simulink model "problem__8"  (R2020b)
settings: Solver=VariableStepAuto  StartTime=0.0  StopTime=10.0  RelTol=1e-3
settings Model: Creator=hp  LastModifiedBy=hp

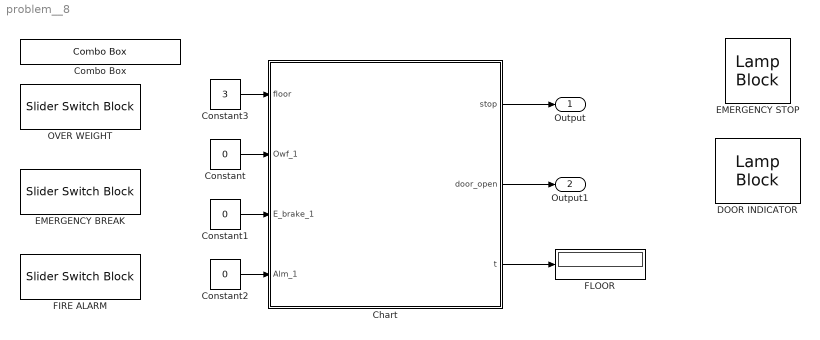
== system problem__8 ==
  Chart : Stateflow chart  TreatAsAtomicUnit=on
  Combo Box : ComboBox  LabelPosition=Hide  SelectedLabel=3rd FLOOR
      settings: Values={{'GROUND FLOOR', '1st FLOOR', '2nd FLOOR', '3rd FLOOR', '4thFLOOR'}, [0 1 2 3 4]}
  Constant : Constant  Value=0
  Constant1 : Constant  Value=0
  Constant2 : Constant  Value=0
  Constant3 : Constant  Value=3
  DOOR INDICATOR : LampBlock
  EMERGENCY BREAK : SliderSwitchBlock
      settings: Values={{'Off', 'On'}, [0 1]}
  EMERGENCY STOP : LampBlock
  FIRE ALARM : SliderSwitchBlock
      settings: Values={{'Off', 'On'}, [0 1]}
  "FLOOR " : Display
  OVER WEIGHT : SliderSwitchBlock
      settings: Values={{'Off', 'On'}, [0 1]}
  Output : Outport
  Output1 : Outport  Port=2
  wires:
  Chart/1(stop) -> Output/1
  Chart/2(door_open) -> Output1/1
  Chart/3(t) -> "FLOOR "/1
  Constant2/1 -> Chart/4(Alm_1)
  Constant/1 -> Chart/2(Owf_1)
  Constant1/1 -> Chart/3(E_brake_1)
  Constant3/1 -> Chart/1(floor)

== stateflow chart problem__8/Chart ==
  state overweight_flag(owf_1) [function]
    (default) -> (junction 160)
    (junction 160) -> (junction 162) [order 1] : [owf_1 ==1]
    (junction 160) -> (junction 167) [order 2]
    (junction 162) -> (junction 165) : {stop=1;}
    (junction 165) -> (junction 167)
    (junction 167) -> (junction 170)
  state LIFT_CONTROL
    state CONTROL
      en:
      i=0;
      i=floor;
      door_open=0;
      overweight_flag(Owf_1);
      fire_alarm(Alm_1);
      emergency_brake(E_brake_1);
      door_open=0;
    state FIRST
      en:
      i=1;
      door_open=1;
      t=1;
      ex:
      door_open=0;
    state SECOND
      en:
      i=2;
      door_open=1;
      t=2;
      ex:
      door_open=0;
    state THIRD
      en:
      i=3;
      door_open=1;
      t=3
      ex:
      door_open=0;
    state FOURTH
      en:
      i=4;
      door_open=1;
      t=4;
      ex:
      door_open=0;
    state GROUND
      en:
      i=0;
      door_open=1;
      t=0;
      ex:
      door_open=0;
    CONTROL -> FOURTH [order 5] : [i==4]
    CONTROL -> THIRD [order 4] : [i==3]
    CONTROL -> SECOND [order 3] : [i==2]
    CONTROL -> FIRST [order 2] : [i==1]
    (default) -> CONTROL
    CONTROL -> GROUND [order 1] : [i==0]
    SECOND -> CONTROL : after(6,sec)[i==6]
    THIRD -> CONTROL : after(6,sec)[i==6]
    GROUND -> CONTROL : after(6,sec)[i==6]
    FIRST -> CONTROL : after(6,sec)[i==6]
    FOURTH -> CONTROL : after(6,sec)[i==6]
  state emergency_brake(e_brake_1) [function]
    (default) -> (junction 190)
    (junction 190) -> (junction 187) [order 1] : [e_brake_1==1]
    (junction 190) -> (junction 196) [order 2]
    (junction 187) -> (junction 193) : {stop=1;}
    (junction 193) -> (junction 196)
    (junction 196) -> (junction 189)
  state fire_alarm(alm_1) [function]
    (default) -> (junction 179)
    (junction 179) -> (junction 176) [order 1] : [alm_1==1]
    (junction 179) -> (junction 185) [order 2]
    (junction 176) -> (junction 182) : {stop=1;}
    (junction 182) -> (junction 185)
    (junction 185) -> (junction 178)
  (default) -> LIFT_CONTROL
  data: owf_1 function_input; e_brake_1 function_input; alm_1 function_input; stop output =0; door_open output; t output; i local; floor input; Owf_1 input; E_brake_1 input; Alm_1 input
